simulink library "FirEven"  (R2022b)
settings: Solver=VariableStepAuto  StartTime=0.0  StopTime=10.0  RelTol=1e-3
libraries: HandyTextFile x4, ITC x2
settings Model: Creator=jb10849  LastModifiedBy=sc48041
settings SolverCC: AlgebraicLoopSolver=TrustRegion
settings DebuggingCC: UnconnectedInputMsg=warning  UnconnectedOutputMsg=warning  UnconnectedLineMsg=warning  SFMachineParentedDataDiag=warning  ArithmeticOperatorsInVariantConditions=warning
settings ModelReferenceCC: EnableRefExpFcnMdlSchedulingChecks=on
settings SFSimCC: SimUseLocalCustomCode=off  CustomCodeUndefinedFunction=UseInterfaceOnly
settings RTWCC: RTWUseLocalCustomCode=off  DLArmComputeVersion=19.05
settings CodeAppCC: StateflowObjectComments=on

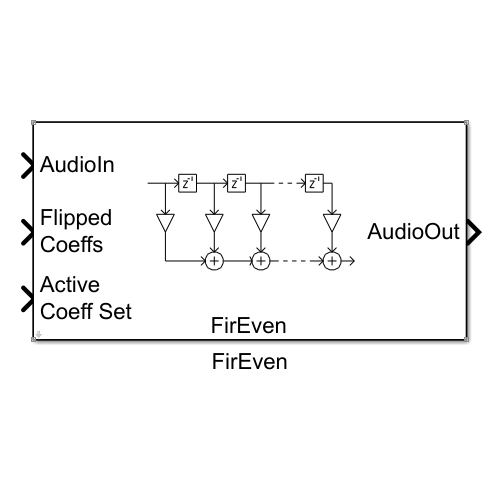
[thumbnail: Simulink's stored preview of the top-level diagram]
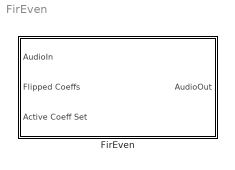
== system FirEven ==
  FirEven : Subsystem  mask{Config=[]}
      mask prompts: Config "FirEvenConfig"
      mask init:
      | blkh=gcbh;
      | Config=BTConfig.Assert(blkh,Config);
      | 
      | Config.Validate();
      | Config.DoMaskInit(blkh);
      mask Display:
      | [path,w,h] = IconFIR_Mask();
      | 
      | port_label('input', 1, 'AudioIn');
      | port_label('input', 2, sprintf('Flipped\nCoeffs'));
      | port_label('input', 3, sprintf('Active\nCoeff Set'));
      | port_label('output', 1, 'AudioOut');
      | 
      | % work in pixels since the icon does not scale
      | pos = get(gcbh,'position');
      | bw = pos(3) - pos(1);
      | bh = pos(4) - pos(2);
      | 
      | % Draw centered icon
      | xAdj = bw/2 - w/2;
      | yAdj = bh/2 - h/2 + 4;
      | for i=1:length(path)
      | %     patch(path(i).x+xAdj, path(i).y+yAdj, path(i).rgb);
      |     plot(path(i).x+xAdj, path(i).y+yAdj);
      | end
      | 
      | % Anchor the corners of the coordinate system
      | patch(0,0,[1 1 1]);
      | patch(bw,bh,[1 1 1]);
      | 
      | % Display some text
      | text(bw/2, 1,'FirEven', ...
      |     'horizontalAlignment','center', ...
      |     'VerticalAlignment','bottom');

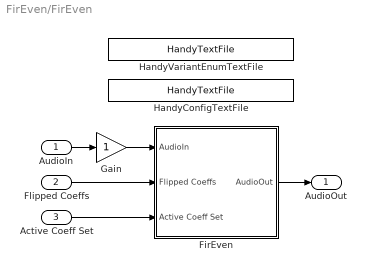
== system FirEven/FirEven ==
  AudioIn : Inport
  Flipped Coeffs : Inport  Port=2
  Active Coeff Set : Inport  Port=3
  FirEven : Subsystem  Variant=on
  Gain : Gain
  HandyConfigTextFile : HandyTextFile/HandyTextFile  TemplateSource=Config  FileSuffix=File  OpenDialogOnLoad=off  UseThisBlockName=off  AddGrandParentNamePrefix=off  TheDefaultText=% $(FILENAME) $(PREFIX) $(SUFFIX)  ShowInLibBrowser=on
      settings: SourceProductName=Bose Talaria
  HandyVariantEnumTextFile : HandyTextFile/HandyTextFile  TemplateSource=VariantEnum  FileSuffix=File  OpenDialogOnLoad=off  UseThisBlockName=off  AddGrandParentNamePrefix=off  TheDefaultText=% $(FILENAME) $(PREFIX) $(SUFFIX)  ShowInLibBrowser=on
      settings: SourceProductName=Bose Talaria
  AudioOut : Outport
  wires:
  AudioIn/1 -> Gain/1
  FirEven/1(AudioOut) -> AudioOut/1
  Flipped Coeffs/1 -> FirEven/2(Flipped Coeffs)
  Active Coeff Set/1 -> FirEven/3(Active Coeff Set)
  Gain/1 -> FirEven/1(AudioIn)

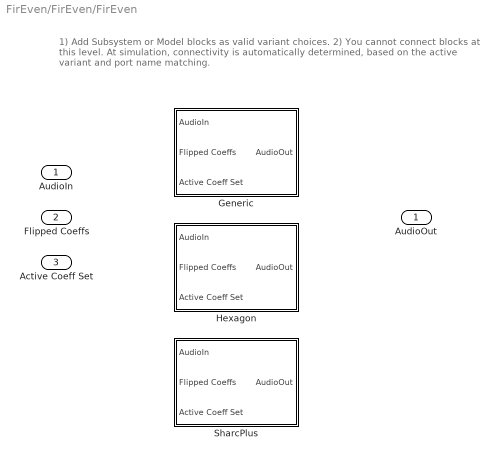
== system FirEven/FirEven/FirEven ==
  note: 1) Add Subsystem or Model blocks as valid variant choices.
      | 2) You cannot connect blocks at this level. At simulation, connectivity is automatically
      | determined, based on the active variant and port name matching.
  AudioIn : Inport
  Flipped Coeffs : Inport  Port=2
  Active Coeff Set : Inport  Port=3
  Generic : Subsystem  VariantControl=(default)
  Hexagon : Subsystem  VariantControl=Config.Variant.StartsWith('Hexagon')
  SharcPlus : Subsystem  VariantControl=Config.Variant.StartsWith('SharcPlus')
  AudioOut : Outport

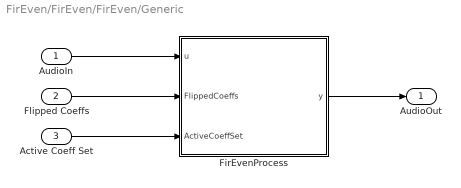
== system FirEven/FirEven/FirEven/Generic ==
  AudioIn : Inport
  Flipped Coeffs : Inport  Port=2
  Active Coeff Set : Inport  Port=3
  FirEvenProcess : MATLAB Function  TreatAsAtomicUnit=on
  AudioOut : Outport
  wires:
  FirEvenProcess/1(y) -> AudioOut/1
  Flipped Coeffs/1 -> FirEvenProcess/2(FlippedCoeffs)
  AudioIn/1 -> FirEvenProcess/1(u)
  Active Coeff Set/1 -> FirEvenProcess/3(ActiveCoeffSet)

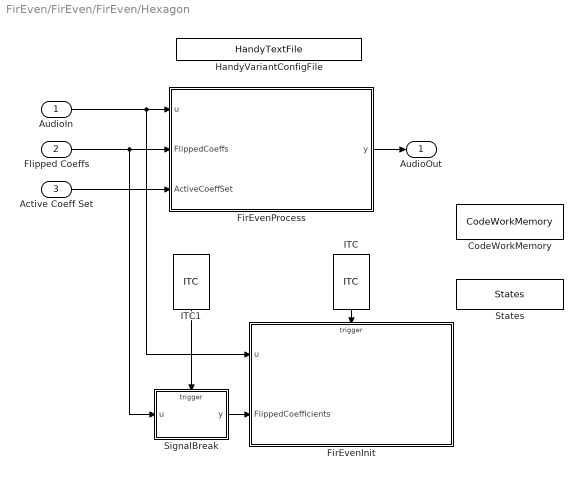
== system FirEven/FirEven/FirEven/Hexagon ==
  AudioIn : Inport
  Flipped Coeffs : Inport  Port=2
  Active Coeff Set : Inport  Port=3
  CodeWorkMemory : DataStoreMemory  DataStoreName=CodeWorkMemory  WriteAfterWriteMsg=warning  InitialValue=uint32(zeros(1,16+4*Config.VariantObj.MaxNumOfThreads+14*Config.VariantObj.MaxNumOfThreads))  ShowAdditionalParam=off  OutDataTypeStr=uint32
  FirEvenInit : MATLAB Function  TreatAsAtomicUnit=on  mask{MaxNumOfThreds=Config.VariantObj.MaxNumOfThreads}
  FirEvenProcess : MATLAB Function  TreatAsAtomicUnit=on
  HandyVariantConfigFile : HandyTextFile/HandyTextFile  TemplateSource=VariantConfig  FileSuffix=Init  OpenDialogOnLoad=off  UseThisBlockName=off  AddGrandParentNamePrefix=on  TheDefaultText=|  ShowInLibBrowser=on
      | % $(FILENAME) Setup model parameters for each "Init" callback (e.g. update diagram)
      | sample_rate_in_hertz = 44100;
      | frame_size = 32;
      | sysin_channel_count = 2;
      settings: SourceProductName=Bose Talaria
  ITC : ITC/ITC
      settings: SourceProductName=Bose Talaria
  ITC1 : ITC/ITC
      settings: SourceProductName=Bose Talaria
  SignalBreak : MATLAB Function  TreatAsAtomicUnit=on
  States : DataStoreMemory  DataStoreName=States  WriteAfterWriteMsg=warning  InitialValue=single(zeros(Config.VariantObj.StateBufferSize,1))  ShowAdditionalParam=off  OutDataTypeStr=single
  AudioOut : Outport
  wires:
  ITC/1 -> FirEvenInit/Trigger
  AudioIn/1 -> FirEvenInit/1(u), FirEvenProcess/1(u)
  Flipped Coeffs/1 -> SignalBreak/1(u), FirEvenProcess/2(FlippedCoeffs)
  Active Coeff Set/1 -> FirEvenProcess/3(ActiveCoeffSet)
  FirEvenProcess/1(y) -> AudioOut/1
  ITC1/1 -> SignalBreak/Trigger
  SignalBreak/1(y) -> FirEvenInit/2(FlippedCoefficients)

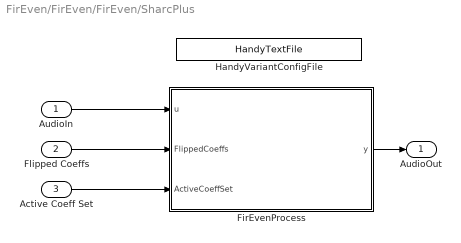
== system FirEven/FirEven/FirEven/SharcPlus ==
  AudioIn : Inport
  Flipped Coeffs : Inport  Port=2
  Active Coeff Set : Inport  Port=3
  FirEvenProcess : MATLAB Function  TreatAsAtomicUnit=on
  HandyVariantConfigFile : HandyTextFile/HandyTextFile  TemplateSource=VariantConfig  FileSuffix=Init  OpenDialogOnLoad=off  UseThisBlockName=off  AddGrandParentNamePrefix=on  TheDefaultText=|  ShowInLibBrowser=on
      | % $(FILENAME) Setup model parameters for each "Init" callback (e.g. update diagram)
      | sample_rate_in_hertz = 44100;
      | frame_size = 32;
      | sysin_channel_count = 2;
      settings: SourceProductName=Bose Talaria
  AudioOut : Outport
  wires:
  FirEvenProcess/1(y) -> AudioOut/1
  Active Coeff Set/1 -> FirEvenProcess/3(ActiveCoeffSet)
  Flipped Coeffs/1 -> FirEvenProcess/2(FlippedCoeffs)
  AudioIn/1 -> FirEvenProcess/1(u)

== matlab function FirEven/FirEven/Hexagon/SignalBreak ==
  data: u input; y output
  events: trigger input FUNCTION_CALL_EVENT
function y = fcn(u)

y = u;

== matlab function FirEven/FirEven/Generic/FirEvenProcess ==
  data: u input; FlippedCoeffs input; y output; ActiveCoeffSet input
function y = FirEvenProcess(u, FlippedCoeffs, ActiveCoeffSet)

[~, NumChannels] = size(u);

y = FirEvenProcessSim(u, NumChannels, ActiveCoeffSet, FlippedCoeffs);

end



% % Extract configuration information from inputs
% [taps, ~] = size(flipped_coeffs);
% [frame_size, num_channels] = size(u);
% 
% % Initialize state variables to zero
% persistent states;
% if isempty(states)
%     states = single(zeros(taps + 2, num_channels));
% end
% % Initialize state index to zero
% persistent state_index;
% if isempty(state_index)
%     state_index = uint32(0);
% end
% 
% % Set correct data types
% filter_length = uint32(taps);
% frame_size = uint32(frame_size);
% num_channels = uint32(num_channels);
% active_coeff_set = uint32(active_coeff_set);
% % Invoking the fir_even function
% y = fir_even(u, frame_size, num_channels, states, filter_length, state_index, active_coeff_set, flipped_coeffs);
% 
% 
% function y = fir_even(u, framesize, numChannels, states, filterLength, stateIndex, activeCoeffSet, coeffs)
% % If target == codegen, generate warning if no CRL found
% coder.replace('-warnifnoreplacement');
% 
% % If running simulation, just use filter()
% % Matlab function takes unflipped coeffs, so coeffs needs to be flipped
% a = 1;
% b = flipud(coeffs);
% [taps, ~] = size(b);
% 
% persistent zi;
% if isempty(zi)
%     zi = single(zeros(taps - 1, numChannels));
% end
% 
% y = single(zeros(size(u)));
% for i = 1:numChannels
%     % Get input, filter coeffs and state for this channel
%     u0 = u(:, i);
%     filterIdx = activeCoeffSet(i) + 1; % add 1 for Matlab indexing
%     coeff = b(:, filterIdx);
%     state = zi(:, i);
%     
%     % Compute output samples and state
%     [y0, state] = filter(coeff, a, u0, state);
%     y(:, i) = y0;
%     
%     % Save state
%     zi(:, i) = state;
% end

== matlab function FirEven/FirEven/Hexagon/FirEvenInit ==
  data: u input; FlippedCoefficients input; CodeWorkMemory data_store_memory; MaxNumOfThreds parameter
  events: trigger input FUNCTION_CALL_EVENT
function FirEvenInit(u, FlippedCoefficients, MaxNumOfThreds)

% Extract configuration information from inputs
[FilterLength, NumFilters] = size(FlippedCoefficients);
[FrameSize, NumChannels] = size(u);

global CodeWorkMemory;

% Simulation 
if(coder.target('MATLAB') || coder.target('Sfun')) 
    return; % No init for simulation code
else
    y = fireven_hexagon_init(uint32(FrameSize), uint32(NumChannels), uint32(NumFilters), uint32(FilterLength), single(FlippedCoefficients), uint32(CodeWorkMemory), uint32(MaxNumOfThreds));
    % NOTE: The CRL mechanism requires an output for the function call,
    % and appears to be optimized out if that return value isn't used. 
    % This is a dummy operation to make sure CRL ends up in generated code
    CodeWorkMemory(1) = y;
end
end

function y = fireven_hexagon_init(frame_size, num_ch, num_of_filters, filter_len, FlippedCoefficients, workMemory, maxNumOfThreds)
coder.replace('-errorifnoreplacement');
[taps, ~] = size(FlippedCoefficients);
y=frame_size + num_ch + num_of_filters + filter_len + taps + workMemory(1);
end

== matlab function FirEven/FirEven/Hexagon/FirEvenProcess ==
  data: u input; y output; FlippedCoeffs input; ActiveCoeffSet input; CodeWorkMemory data_store_memory; States data_store_memory
function y = FirEvenProcess(u, FlippedCoeffs, ActiveCoeffSet)

% Extract configuration information from inputs
[FilterLength, ~] = size(FlippedCoeffs);
[FrameSize, NumChannels] = size(u);

global CodeWorkMemory;
global States;

% Initialize variables
% persistent States;
% if isempty(States)
%     States = single(zeros(FilterLength + FrameSize*2 + 2, NumChannels));
% end

% Set correct data types
FilterLength = uint32(FilterLength);
FrameSize = uint32(FrameSize);
ActiveCoeffSet = uint32(ActiveCoeffSet);


if(coder.target('MATLAB') || coder.target('Sfun')) 
    % FIREVEN SIMULATION
    y = FirEvenProcessSim(u, NumChannels, ActiveCoeffSet, FlippedCoeffs);
else
    % FIR EVEN HEXAGON
    if (FilterLength > FrameSize)
        y = fireven_hexagon_process_mt(single(u), uint32(ActiveCoeffSet), single(States), uint32(CodeWorkMemory));
    else
        y = fireven_hexagon_process_lt(single(u), uint32(ActiveCoeffSet), single(States), uint32(CodeWorkMemory));
    end
end    
end
  

function y = fireven_hexagon_process_mt(u, ActiveCoeffSet, States, WorkMemory)
coder.replace('-errorifnoreplacement');
[fs, num_ch]  = size(u);
y = single(zeros(fs, num_ch));
end

function y = fireven_hexagon_process_lt(u, ActiveCoeffSet, States, WorkMemory)
coder.replace('-errorifnoreplacement');
[fs, num_ch]  = size(u);
y = single(zeros(fs, num_ch));
end

== matlab function FirEven/FirEven/SharcPlus/FirEvenProcess ==
  data: u input; y output; FlippedCoeffs input; ActiveCoeffSet input
function y = FirEvenProcess(u, FlippedCoeffs, ActiveCoeffSet)

% Extract configuration information from inputs
[FilterLength, ~] = size(FlippedCoeffs);
[FrameSize, NumChannels] = size(u);

% Initialize variables
persistent States;
if isempty(States)
    States = single(zeros(FilterLength + FrameSize + 2, NumChannels));
end

% Initialize state index to zero
persistent StateIndex;
if isempty(StateIndex)
    StateIndex = uint32(0);
end


if(coder.target('MATLAB') || coder.target('Sfun')) 
    % FIREVEN SIMULATION
    y = FirEvenProcessSim(u, NumChannels, ActiveCoeffSet, FlippedCoeffs);
else
    y = fir_even(single(u), uint32(FrameSize), uint32(NumChannels), single(States), ...
        uint32(FilterLength), uint32(StateIndex), uint32(ActiveCoeffSet), single(FlippedCoeffs));
end

end

function y = fir_even(u, FrameSize, NumChannels, States, FilterLength, StateIndex, ActiveCoeffSet, Coeffs)
% If target == codegen, generate warning if no CRL found
coder.replace('-warnifnoreplacement');
y = single(zeros(FrameSize, NumChannels));
end
